simulink model "b2c"  (R2018a)
settings: Solver=VariableStepAuto  StartTime=0.0  StopTime=100  RelTol=1e-3
libraries: simulink x3
settings Model: Creator=Huy  LastModifiedBy=Huy

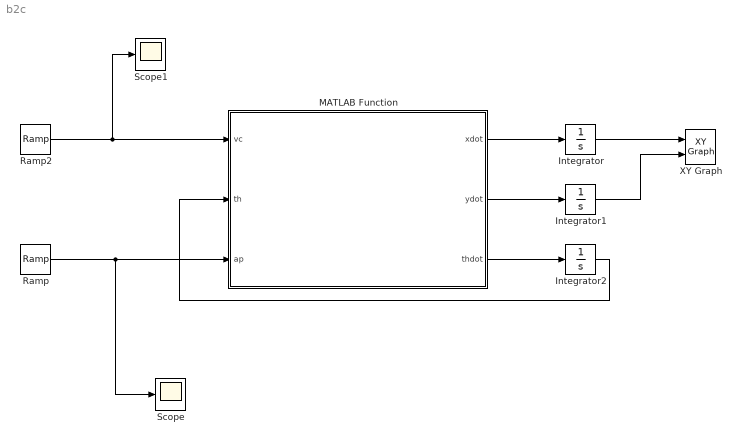
== system b2c ==
  Integrator : Integrator
  Integrator1 : Integrator
  Integrator2 : Integrator
  MATLAB Function : MATLAB Function  TreatAsAtomicUnit=on
  Ramp : simulink/Sources/Ramp  slope=1  start=0  InitialOutput=0
  Ramp2 : simulink/Sources/Ramp  slope=1  start=0  InitialOutput=0
  Scope : Scope
  Scope1 : Scope
  XY Graph : simulink/Sinks/XY Graph  xmin=-1  xmax=1  ymin=-8  ymax=1  st=1
  wires:
  MATLAB Function/1(xdot) -> Integrator/1
  MATLAB Function/2(ydot) -> Integrator1/1
  MATLAB Function/3(thdot) -> Integrator2/1
  Integrator/1 -> XY Graph/1
  Integrator1/1 -> XY Graph/2
  Ramp/1 -> Scope/1, MATLAB Function/3(ap)
  Integrator2/1 -> MATLAB Function/2(th)
  Ramp2/1 -> Scope1/1, MATLAB Function/1(vc)

== matlab function b2c/MATLAB Function ==
  data: vc input; xdot output; th input; ap input; ydot output; thdot output
function [xdot,ydot,thdot] = tricycle (vc,th,ap)
vmax = 0.36; %van toc cuc dai cua robot 
amax = 0.28; %gia toc cuc dai cua robot
apmax = (pi/4)*180/pi %goc lai cuc dai cua robot = 45 do 
wmax = 0.30; % van toc goc cuc dai cua robot 
G = 13;%Nhom
d = sqrt(2.5 + 0.1*G);
xdot = vc*cos(th)*cos(ap); %van toc theo phUong x
ydot = vc*sin(th)*cos(ap);  %van toc theo phuong y
thdot = vc/d *sin(ap); %van toc goc
%vc = v/cos(alpha)
%vcmax = 0.36 /sqrt(2)/2 = 0.509 m/s;
%vcmin = 0 m/s;
